simulink model "part1"  (R2014a)
settings: Solver=ode45  StartTime=0.0  StopTime=10.0  RelTol=1e-3
settings Model: Creator=SuperUser  LastModifiedBy=SuperUser

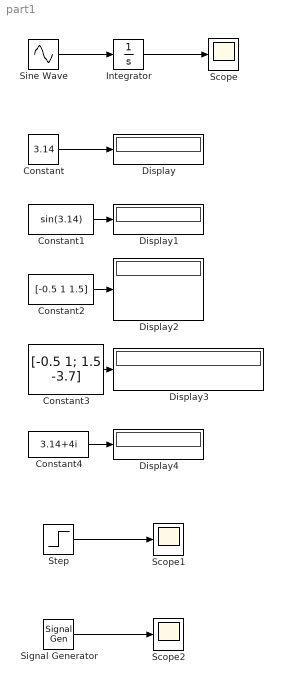
== system part1 ==
  Constant : Constant  Value=3.14
  Constant1 : Constant  Value=sin(3.14)
  Constant2 : Constant  Value=[-0.5 1 1.5]
  Constant3 : Constant  Value=[-0.5 1; 1.5 -3.7]
  Constant4 : Constant  Value=3.14+4i
  Display{,1..4} (5 alike) : Display
  Integrator : Integrator
  Scope : Scope
  Scope1 : Scope
  Scope2 : Scope
      settings: SaveName=ScopeData2
  Signal Generator : SignalGenerator  WaveForm=square  Units=rad/sec
  Sine Wave : Sin  SampleTime=0
  Step : Step  SampleTime=0
  wires:
  Sine Wave/1 -> Integrator/1
  Integrator/1 -> Scope/1
  Constant/1 -> Display/1
  Constant1/1 -> Display1/1
  Constant2/1 -> Display2/1
  Constant3/1 -> Display3/1
  Constant4/1 -> Display4/1
  Step/1 -> Scope1/1
  Signal Generator/1 -> Scope2/1
